simulink library "PC_Simulator_Lib"  (Simulink 8.2)
settings: Solver=ode45  StartTime=0.0  StopTime=10.0  RelTol=1e-3
values from neighbouring files (symbols this model uses):
  data = [r1 r2 r3 r4 L1 L2 L3 L4]    [strasse_Bedatung_HNI_ITI.m]
  distSameLane = 60    [InitialisationsEnv.m]
  eng_speed = [0 60 120 180 240 300 360 420 480 540 600 660 ... (101 elements, 1x101)]    [engine_table.mat]    (also in motor_parameter_calc.m = omega)
  Heading_init = 0    [Start.m]
  inertiaLateral = 25*(radiusWheel)^2    (= 4.129024)    [Start.m]
  laneWidth = 3.6    [InitialisationsEnv.m]    (also in strasse_Bedatung_HNI_ITI.m)
  omega_engine = [0.000000 150.000000 500.000000 1000.000000 1500.000000 2000.000000 2500.000000 3000.000000 3500.000000 4000.000000 4500.000000 5000.000000 5500.000000 6000.000000]    [friction_tables.m]
  omega_max = 6000    [engine_table.mat]    (also in motor_parameter_calc.m)
  omega_wheel = [0 20 40 60 80 100 122 143.7 164]    [friction_tables.m]
  para_Fellow_8_Points = ADAS.Fellow_8_Points    [ADAS_parameters.m]
  position_start_x = [x1 x2 x3 x4 x5 x6 x7]    [strasse_Bedatung_HNI_ITI.m]
  position_start_y = [y1 y2 y3 y4 y5 y6 y7]    [strasse_Bedatung_HNI_ITI.m]
  rad3rdLine = 57.2    [InitialisationsEnv.m]    (also in strasse_Bedatung_HNI_ITI.m)
  radiusWheel = 16*2.54/100    (= 0.4064)    [Start.m]
  s_values = [S1 S2 S3 S4 S5 S6 S7]    [strasse_Bedatung_HNI_ITI.m]
  segmentLimits = [segment1EndThirdLine                   segment2EndThirdLine                   segment3EndThirdLine                   segment4EndThirdLine                   segment5EndThirdLine                   segment6EndThirdLine                   segment7EndThirdLine                   segment8EndThirdLine                   ]    [InitialisationsEnv.m]    (also in strasse_Bedatung_HNI_ITI.m)
  setPosT = [-1.8 -5.4 -1.8 -5.4 -1.8 -5.4 -1.8 -5.4 -1.8 -5.4]    [InitialisationsEnv.m]
  torque = [297.089227105 300.997600937 304.800343044 308.497453426 312.088932082 315.574779014 318.95499422 322.229577701 325.398529457 328.461849487 331.419537793 334.271594373 ... (101 elements, 1x101)]    [engine_table.mat]    (also in motor_parameter_calc.m = g)
  Torque_lost = [0.000000 -8.777780 -15.000000 -26.800000 -29.600000 -32.700000 -35.900000 -39.300000 -42.800000 -46.500000 -50.300000 -54.300000 -58.500000 -62.800000 ]*0.6    [friction_tables.m]
  Torque_lost_wheel = [0.8 0.8 0.75 0.7 0.4 0.3 0.2 0.07 0.07]*0.2    [friction_tables.m]
  X_init = 0    [Start.m]
  Y_init = 1.8    [Start.m]
  Z_init = 0    [Start.m]
undefined symbols (not defined in the file or in its folder): Acc_Pedal, ADAS, Brake_Pedal, Joystick, Newton, Para, Raphson, Standard_Devices, Steering_Wheel_Angle, UDP_Protocol
libraries: simulink x43, rtwinlib x7, dspnetwork x2, simulink_extras x1, vrlib x1
(part 1 of 13)
settings Model: Creator=fahim  LastModifiedBy=fahim

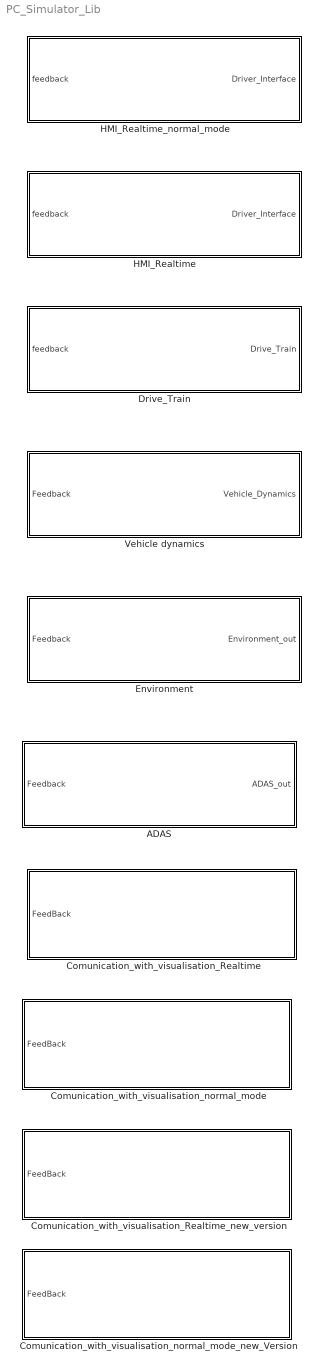
== system PC_Simulator_Lib ==
  ADAS : Subsystem
  Comunication_with_visualisation_Realtime : Subsystem
  Comunication_with_visualisation_Realtime_new_version : Subsystem
  Comunication_with_visualisation_normal_mode : Subsystem
  Comunication_with_visualisation_normal_mode_new_Version : Subsystem
  Drive_Train : Subsystem
  Environment : Subsystem
  HMI_Realtime : Subsystem
  HMI_Realtime_normal_mode : Subsystem
  Vehicle dynamics : Subsystem

== system PC_Simulator_Lib/ADAS ==
  Feedback : Inport
  Bus Creator : BusCreator  Inputs=9
  Bus Creator1 : BusCreator
  Bus Creator2 : BusCreator
  Bus Selector : BusSelector  OutputSignals=Execution_ADAS.actions_on_vehicle.Acc_Pedal[norm],Execution_ADAS.actions_on_vehicle.Brake_Pedal[norm],Execution_ADAS.actions_on_vehicle.Steering_Wheel_Angle[norm],Decision_Making_ADAS.Enable_Lateral_Controller,Unser_Interface_ADAS.ACC.ACC_Set_Speed[m|s],Decision_Making_ADAS.level_of_danger_front[0-3],Decision_Making_ADAS.Brake_distance[m],Sensors_ADAS.Sensors_Front_Out.Distance[m],Unser_Interface_ADAS.ACC.ACC_State,Unser_Interface_ADAS.Pilotiertes_Fahren.Pilotiertes_Fahren_State,Unser_Interface_ADAS.Emergency_Brake.Emergency_Brake_State,Unser_Interface_ADAS.Emergency_Steering.Emergency_Steering_State
  Decision_Making_ADAS : Subsystem
  Execution_ADAS : Subsystem
  Sensors_ADAS : Subsystem
  Unser_Interface_ADAS : Subsystem
  ADAS_out : Outport
  wires:
  Bus Selector/8 -> Bus Creator/8  "<Distance[m]>"
  Bus Selector/7 -> Bus Creator/7  "<Brake_distance[m]>"
  Bus Selector/6 -> Bus Creator/6  "<level_of_danger_front[0-3]>"
  Bus Selector/5 -> Bus Creator/5  "<ACC_Set_Speed[m|s]>"
  Bus Creator/1 -> ADAS_out/1  "ADAS"
  Unser_Interface_ADAS/1(UnserInterface_ADAS) -> Bus Creator1/1  "Unser_Interface_ADAS"
  Sensors_ADAS/1(Sensors_ADAS) -> Bus Creator1/2  "Sensors_ADAS"
  Decision_Making_ADAS/1(Decision_ADAS) -> Bus Creator1/3  "Decision_Making_ADAS"
  Execution_ADAS/1(Execution_ADAS) -> Bus Creator1/4  "Execution_ADAS"
  Bus Creator1/1 -> Sensors_ADAS/1(Feedback_ADAS), Unser_Interface_ADAS/1(Feedback_ADAS), Decision_Making_ADAS/1(Feedback_ADAS), Execution_ADAS/1(Feedback_ADAS), Bus Selector/1
  Feedback/1 -> Unser_Interface_ADAS/2(Feedback_Simulationsumgebung), Sensors_ADAS/2(Feedback_Simulationsumgebung), Execution_ADAS/2(Feedback_Simulationsumgebung), Decision_Making_ADAS/2(Feedback_Simulationsumgebung)
  Bus Selector/1 -> Bus Creator/1  "<Acc_Pedal[norm]>"
  Bus Selector/2 -> Bus Creator/2  "<Brake_Pedal[norm]>"
  Bus Selector/3 -> Bus Creator/3  "<Steering_Wheel_Angle[norm]>"
  Bus Creator2/1 -> Bus Creator/9  "ADAS_Systems_States"
  Bus Selector/9 -> Bus Creator2/1  "<ACC_State>"
  Bus Selector/10 -> Bus Creator2/2  "<Pilotiertes_Fahren_State>"
  Bus Selector/11 -> Bus Creator2/3  "<Emergency_Brake_State>"
  Bus Selector/12 -> Bus Creator2/4  "<Emergency_Steering_State>"
  Bus Selector/4 -> Bus Creator/4  "<Enable_Lateral_Controller>"

== system PC_Simulator_Lib/Comunication_with_visualisation_Realtime ==
  FeedBack : Inport
  Bus Selector : BusSelector  OutputSignals=Vehicle_Dynamics.position_CoG,Vehicle_Dynamics.Oriantation_CoG
  Bus Selector1 : BusSelector  OutputSignals=ADAS.Steering_Wheel_Angle[norm]
  Bus Selector2 : BusSelector  OutputSignals=Drive_Train.Omega_Engine[rad|s]
  Bus Selector3 : BusSelector  OutputSignals=Vehicle_Dynamics.Vx_COG[m|s]
  Embedded MATLAB Function : MATLAB Function  TreatAsAtomicUnit=on
  Gain : Gain  Gain=180/pi
  Gain1 : Gain  Gain=0.5
  Gain2 : Gain  Gain=-450
  Maping_Block : Subsystem
  Packet Output : rtwinlib/Packet Output  SampleTime=0.001  MaxMissedTicks=[]  ShowMissedTicks=off  YieldWhenWaiting=on  DrvName=Standard_Devices/UDP_Protocol  DrvAddress=15005  DrvOptions=[2213172829 15005]  PacketSize=1064  DataTypes='1064*uint8'  ShowReady=off  ShowError=off  PacketID=1  ByteOrder=1  InitialValue=[]  FinalValue=[]
      settings: AttributesFormatString=Standard Devices\nUDP Protocol [3A9Dh]
  Subsystem : Subsystem
  Subsystem1 : Subsystem
  Subsystem2 : Subsystem
  Subsystem3 : Subsystem
  Subsystem4 : Subsystem
  Subsystem5 : Subsystem
  wires:
  Embedded MATLAB Function/1(y) -> Packet Output/1
  Bus Selector/2 -> Subsystem1/1(In1)  "<Oriantation_CoG>"
  Bus Selector/1 -> Subsystem/1(In1)  "<position_CoG>"
  Subsystem/1(Out1) -> Maping_Block/1(VUT_Position_xyz[m])
  Subsystem1/1(Out1) -> Gain/1
  Subsystem2/2(Vehicle_1_Vector) -> Maping_Block/8(Vehicle_1_Vector)
  Subsystem2/3(Vehicle_2_Vector) -> Maping_Block/9(Vehicle_2_Vector)
  Subsystem2/4(Vehicle_3_Vector) -> Maping_Block/10(Vehicle_3_Vector)
  Subsystem2/5(Vehicle_4_Vector3) -> Maping_Block/11(Vehicle_4_Vector)
  Subsystem2/6(Vehicle_5_Vector) -> Maping_Block/12(Vehicle_5_Vector)
  Subsystem2/7(Vehicle_6_Vector) -> Maping_Block/13(Vehicle_6_Vector)
  Subsystem2/8(Vehicle_7_Vector) -> Maping_Block/14(Vehicle_7_Vector)
  Subsystem2/9(Vehicle_8_Vector) -> Maping_Block/15(Vehicle_8_Vector)
  Subsystem2/10(Vehicle_9_Vector) -> Maping_Block/16(Vehicle_9_Vector)
  Subsystem2/11(Vehicle_10_Vector) -> Maping_Block/17(Vehicle_10_Vector)
  Subsystem2/12(Vehicle_11_Vector) -> Maping_Block/18(Vehicle_11_Vector)
  Subsystem2/13(Vehicle_12_Vector) -> Maping_Block/19(Vehicle_12_Vector)
  Subsystem2/14(Vehicle_13_Vector) -> Maping_Block/20(Vehicle_13_Vector)
  Subsystem2/15(Vehicle_14_Vector) -> Maping_Block/21(Vehicle_14_Vector)
  Gain/1 -> Maping_Block/2(VUT_Oriantation_xyz[deg])
  Subsystem5/1(Out1) -> Maping_Block/4(VUT_Front_Wheels_Steering_Angle[deg])
  Subsystem2/1(Enablble_Fellow_Vehicles[bool]) -> Maping_Block/7(Enable_Vehicles_Vector_14[bool])
  Maping_Block/1(To_UDP) -> Embedded MATLAB Function/1(u)
  Subsystem3/1(Out1) -> Maping_Block/6(VUT_Engine_rpm)
  Bus Selector1/1 -> Gain2/1  "<Steering_Wheel_Angle[norm]>"
  Gain1/1 -> Maping_Block/3(VUT_Steering_Wheel_Angle[deg])
  Gain2/1 -> Gain1/1
  Bus Selector3/1 -> Subsystem4/1(In1)  "<Vx_COG[m|s]>"
  Subsystem4/1(Out1) -> Maping_Block/5(VUT_Wheels_Rotation_Angle[rad])
  FeedBack/1 -> Bus Selector/1, Bus Selector3/1, Bus Selector2/1, Subsystem2/1(FeedBack), Subsystem5/1(In1), Bus Selector1/1
  Bus Selector2/1 -> Subsystem3/1(In1)  "<Omega_Engine[rad|s]>"

== system PC_Simulator_Lib/Comunication_with_visualisation_Realtime_new_version ==
  FeedBack : Inport
  Bus Selector : BusSelector  OutputSignals=Vehicle_Dynamics.position_CoG,Vehicle_Dynamics.Oriantation_CoG
  Bus Selector1 : BusSelector  OutputSignals=ADAS.Steering_Wheel_Angle[norm]
  Bus Selector2 : BusSelector  OutputSignals=Drive_Train.Omega_Engine[rad|s]
  Bus Selector3 : BusSelector  OutputSignals=Vehicle_Dynamics.Vx_COG[m|s]
  Bus Selector4 : BusSelector  OutputSignals=ADAS.ACC_Set_Speed[m|s],ADAS.level_of_danger_front[0-3]
  Embedded MATLAB Function : MATLAB Function  TreatAsAtomicUnit=on
  Gain : Gain  Gain=180/pi
  Gain2 : Gain  Gain=-450
  Ground : Ground
  Ground1 : Ground
  Ground2 : Ground
  Maping_Block : Subsystem
  Packet Output : rtwinlib/Packet Output  SampleTime=0.001  MaxMissedTicks=[]  ShowMissedTicks=off  YieldWhenWaiting=on  DrvName=Standard_Devices/UDP_Protocol  DrvAddress=15005  DrvOptions=[2213172829 15005]  PacketSize=1120  DataTypes='1120*uint8'  ShowReady=off  ShowError=off  PacketID=1  ByteOrder=1  InitialValue=[]  FinalValue=[]
      settings: AttributesFormatString=Standard Devices\nUDP Protocol [3A9Dh]
  Subsystem : Subsystem
  Subsystem1 : Subsystem
  Subsystem2 : Subsystem
  Subsystem3 : Subsystem
  Subsystem4 : Subsystem
  Subsystem5 : Subsystem
  Subsystem6 : Subsystem
  scaling_factor : Gain  Gain=0.4457
  scaling_factor1 : Gain  Gain=1/8
  scaling_factor2 : Gain  Gain=3.6
  scaling_factor3 : Gain  Gain=3.6
  wires:
  scaling_factor3/1 -> Maping_Block/23(User_Set_Speed[km|h])
  Bus Selector4/2 -> Maping_Block/24(LED_Front_State)  "<level_of_danger_front[0-3]>"
  Bus Selector4/1 -> scaling_factor3/1  "<ACC_Set_Speed[m|s]>"
  Subsystem6/1(Out1) -> Maping_Block/22(Activated_ADAS)
  Ground2/1 -> Maping_Block/27(LED_Left_State)
  Ground1/1 -> Maping_Block/26(LED_Right_State)
  Ground/1 -> Maping_Block/25(LED_Back_State)
  scaling_factor2/1 -> scaling_factor/1
  scaling_factor/1 -> Maping_Block/21(VUT_Speed[km|h])
  Bus Selector2/1 -> Subsystem3/1(In1)  "<Omega_Engine[rad|s]>"
  FeedBack/1 -> Bus Selector1/1, Subsystem5/1(In1), Bus Selector3/1, Bus Selector2/1, Subsystem6/1(In1), Bus Selector4/1, Subsystem2/1(FeedBack), Bus Selector/1
  Subsystem4/1(Out1) -> Maping_Block/5(VUT_Wheels_Rotation_Angle[rad])
  Bus Selector3/1 -> Subsystem4/1(In1), scaling_factor2/1  "<Vx_COG[m|s]>"
  Gain2/1 -> scaling_factor1/1
  scaling_factor1/1 -> Maping_Block/3(VUT_Steering_Wheel_Angle[deg])
  Bus Selector1/1 -> Gain2/1  "<Steering_Wheel_Angle[norm]>"
  Subsystem3/1(Out1) -> Maping_Block/6(VUT_Engine_rpm)
  Maping_Block/1(To_UDP) -> Embedded MATLAB Function/1(u)
  Subsystem5/1(Out1) -> Maping_Block/4(VUT_Front_Wheels_Steering_Angle[deg])
  Gain/1 -> Maping_Block/2(VUT_Oriantation_xyz[deg])
  Subsystem2/14(Vehicle_14_Vector) -> Maping_Block/20(Vehicle_14_Vector)
  Subsystem2/13(Vehicle_13_Vector) -> Maping_Block/19(Vehicle_13_Vector)
  Subsystem2/12(Vehicle_12_Vector) -> Maping_Block/18(Vehicle_12_Vector)
  Subsystem2/11(Vehicle_11_Vector) -> Maping_Block/17(Vehicle_11_Vector)
  Subsystem2/10(Vehicle_10_Vector) -> Maping_Block/16(Vehicle_10_Vector)
  Subsystem2/9(Vehicle_9_Vector) -> Maping_Block/15(Vehicle_9_Vector)
  Subsystem2/8(Vehicle_8_Vector) -> Maping_Block/14(Vehicle_8_Vector)
  Subsystem2/7(Vehicle_7_Vector) -> Maping_Block/13(Vehicle_7_Vector)
  Subsystem2/6(Vehicle_6_Vector) -> Maping_Block/12(Vehicle_6_Vector)
  Subsystem2/5(Vehicle_5_Vector) -> Maping_Block/11(Vehicle_5_Vector)
  Subsystem2/4(Vehicle_4_Vector3) -> Maping_Block/10(Vehicle_4_Vector)
  Subsystem2/3(Vehicle_3_Vector) -> Maping_Block/9(Vehicle_3_Vector)
  Subsystem2/2(Vehicle_2_Vector) -> Maping_Block/8(Vehicle_2_Vector)
  Subsystem2/1(Vehicle_1_Vector) -> Maping_Block/7(Vehicle_1_Vector)
  Subsystem1/1(Out1) -> Gain/1
  Subsystem/1(Out1) -> Maping_Block/1(VUT_Position_xyz[m])
  Bus Selector/1 -> Subsystem/1(In1)  "<position_CoG>"
  Bus Selector/2 -> Subsystem1/1(In1)  "<Oriantation_CoG>"
  Embedded MATLAB Function/1(y) -> Packet Output/1

== system PC_Simulator_Lib/Comunication_with_visualisation_normal_mode ==
  FeedBack : Inport
  Bus Selector : BusSelector  OutputSignals=Vehicle_Dynamics.position_CoG,Vehicle_Dynamics.Oriantation_CoG
  Bus Selector1 : BusSelector  OutputSignals=ADAS.Steering_Wheel_Angle[norm]
  Bus Selector2 : BusSelector  OutputSignals=Drive_Train.Omega_Engine[rad|s]
  Bus Selector3 : BusSelector  OutputSignals=Vehicle_Dynamics.Vx_COG[m|s]
  Embedded MATLAB Function : MATLAB Function  TreatAsAtomicUnit=on
  Gain : Gain  Gain=180/pi
  Gain1 : Gain  Gain=0.5
  Gain2 : Gain  Gain=-450
  Maping_Block : Subsystem
  Subsystem : Subsystem
  Subsystem1 : Subsystem
  Subsystem2 : Subsystem
  Subsystem3 : Subsystem
  Subsystem4 : Subsystem
  Subsystem5 : Subsystem
  UDP Send : dspnetwork/UDP Send  remoteURL='131.234.86.93'  remotePort=15005  localURL='0.0.0.0'  localPortSource=Automatically determine  localPort=-1  sampletime=-1  separateLengthPort=0
  wires:
  Embedded MATLAB Function/1(y) -> UDP Send/1
  Bus Selector/2 -> Subsystem1/1(In1)  "<Oriantation_CoG>"
  Bus Selector/1 -> Subsystem/1(In1)  "<position_CoG>"
  Subsystem/1(Out1) -> Maping_Block/1(VUT_Position_xyz[m])
  Subsystem1/1(Out1) -> Gain/1
  Subsystem2/2(Vehicle_1_Vector) -> Maping_Block/8(Vehicle_1_Vector)
  Subsystem2/3(Vehicle_2_Vector) -> Maping_Block/9(Vehicle_2_Vector)
  Subsystem2/4(Vehicle_3_Vector) -> Maping_Block/10(Vehicle_3_Vector)
  Subsystem2/5(Vehicle_4_Vector3) -> Maping_Block/11(Vehicle_4_Vector)
  Subsystem2/6(Vehicle_5_Vector) -> Maping_Block/12(Vehicle_5_Vector)
  Subsystem2/7(Vehicle_6_Vector) -> Maping_Block/13(Vehicle_6_Vector)
  Subsystem2/8(Vehicle_7_Vector) -> Maping_Block/14(Vehicle_7_Vector)
  Subsystem2/9(Vehicle_8_Vector) -> Maping_Block/15(Vehicle_8_Vector)
  Subsystem2/10(Vehicle_9_Vector) -> Maping_Block/16(Vehicle_9_Vector)
  Subsystem2/11(Vehicle_10_Vector) -> Maping_Block/17(Vehicle_10_Vector)
  Subsystem2/12(Vehicle_11_Vector) -> Maping_Block/18(Vehicle_11_Vector)
  Subsystem2/13(Vehicle_12_Vector) -> Maping_Block/19(Vehicle_12_Vector)
  Subsystem2/14(Vehicle_13_Vector) -> Maping_Block/20(Vehicle_13_Vector)
  Subsystem2/15(Vehicle_14_Vector) -> Maping_Block/21(Vehicle_14_Vector)
  Gain/1 -> Maping_Block/2(VUT_Oriantation_xyz[deg])
  Subsystem5/1(Out1) -> Maping_Block/4(VUT_Front_Wheels_Steering_Angle[deg])
  Subsystem2/1(Enablble_Fellow_Vehicles[bool]) -> Maping_Block/7(Enable_Vehicles_Vector_14[bool])
  Maping_Block/1(To_UDP) -> Embedded MATLAB Function/1(u)
  Subsystem3/1(Out1) -> Maping_Block/6(VUT_Engine_rpm)
  Bus Selector1/1 -> Gain2/1  "<Steering_Wheel_Angle[norm]>"
  Gain1/1 -> Maping_Block/3(VUT_Steering_Wheel_Angle[deg])
  Gain2/1 -> Gain1/1
  Bus Selector3/1 -> Subsystem4/1(In1)  "<Vx_COG[m|s]>"
  Subsystem4/1(Out1) -> Maping_Block/5(VUT_Wheels_Rotation_Angle[rad])
  FeedBack/1 -> Bus Selector/1, Bus Selector3/1, Bus Selector2/1, Subsystem2/1(FeedBack), Subsystem5/1(In1), Bus Selector1/1
  Bus Selector2/1 -> Subsystem3/1(In1)  "<Omega_Engine[rad|s]>"

== system PC_Simulator_Lib/Comunication_with_visualisation_normal_mode_new_Version ==
  FeedBack : Inport
  Bus Selector : BusSelector  OutputSignals=Vehicle_Dynamics.position_CoG,Vehicle_Dynamics.Oriantation_CoG
  Bus Selector1 : BusSelector  OutputSignals=ADAS.Steering_Wheel_Angle[norm]
  Bus Selector2 : BusSelector  OutputSignals=Drive_Train.Omega_Engine[rad|s]
  Bus Selector3 : BusSelector  OutputSignals=Vehicle_Dynamics.Vx_COG[m|s]
  Bus Selector4 : BusSelector  OutputSignals=ADAS.ACC_Set_Speed[m|s],ADAS.level_of_danger_front[0-3]
  Embedded MATLAB Function : MATLAB Function  TreatAsAtomicUnit=on
  Gain : Gain  Gain=180/pi
  Gain2 : Gain  Gain=-450
  Ground : Ground
  Ground1 : Ground
  Ground2 : Ground
  Maping_Block : Subsystem
  Subsystem : Subsystem
  Subsystem1 : Subsystem
  Subsystem2 : Subsystem
  Subsystem3 : Subsystem
  Subsystem4 : Subsystem
  Subsystem5 : Subsystem
  Subsystem6 : Subsystem
  UDP Send : dspnetwork/UDP Send  remoteURL='131.234.86.93'  remotePort=15005  localURL='0.0.0.0'  localPortSource=Automatically determine  localPort=-1  sampletime=-1  separateLengthPort=0
  scaling_factor : Gain  Gain=0.4457
  scaling_factor1 : Gain  Gain=1/8
  scaling_factor2 : Gain  Gain=3.6
  scaling_factor3 : Gain  Gain=3.6
  wires:
  scaling_factor3/1 -> Maping_Block/23(User_Set_Speed[km|h])
  Bus Selector4/2 -> Maping_Block/24(LED_Front_State)  "<level_of_danger_front[0-3]>"
  Bus Selector4/1 -> scaling_factor3/1  "<ACC_Set_Speed[m|s]>"
  Subsystem6/1(Out1) -> Maping_Block/22(Activated_ADAS)
  Ground2/1 -> Maping_Block/27(LED_Left_State)
  Ground1/1 -> Maping_Block/26(LED_Right_State)
  Ground/1 -> Maping_Block/25(LED_Back_State)
  scaling_factor2/1 -> scaling_factor/1
  scaling_factor/1 -> Maping_Block/21(VUT_Speed[km|h])
  Bus Selector2/1 -> Subsystem3/1(In1)  "<Omega_Engine[rad|s]>"
  FeedBack/1 -> Bus Selector1/1, Subsystem5/1(In1), Bus Selector3/1, Bus Selector2/1, Subsystem6/1(In1), Bus Selector4/1, Subsystem2/1(FeedBack), Bus Selector/1
  Subsystem4/1(Out1) -> Maping_Block/5(VUT_Wheels_Rotation_Angle[rad])
  Bus Selector3/1 -> Subsystem4/1(In1), scaling_factor2/1  "<Vx_COG[m|s]>"
  Gain2/1 -> scaling_factor1/1
  scaling_factor1/1 -> Maping_Block/3(VUT_Steering_Wheel_Angle[deg])
  Bus Selector1/1 -> Gain2/1  "<Steering_Wheel_Angle[norm]>"
  Subsystem3/1(Out1) -> Maping_Block/6(VUT_Engine_rpm)
  Maping_Block/1(To_UDP) -> Embedded MATLAB Function/1(u)
  Subsystem5/1(Out1) -> Maping_Block/4(VUT_Front_Wheels_Steering_Angle[deg])
  Gain/1 -> Maping_Block/2(VUT_Oriantation_xyz[deg])
  Subsystem2/14(Vehicle_14_Vector) -> Maping_Block/20(Vehicle_14_Vector)
  Subsystem2/13(Vehicle_13_Vector) -> Maping_Block/19(Vehicle_13_Vector)
  Subsystem2/12(Vehicle_12_Vector) -> Maping_Block/18(Vehicle_12_Vector)
  Subsystem2/11(Vehicle_11_Vector) -> Maping_Block/17(Vehicle_11_Vector)
  Subsystem2/10(Vehicle_10_Vector) -> Maping_Block/16(Vehicle_10_Vector)
  Subsystem2/9(Vehicle_9_Vector) -> Maping_Block/15(Vehicle_9_Vector)
  Subsystem2/8(Vehicle_8_Vector) -> Maping_Block/14(Vehicle_8_Vector)
  Subsystem2/7(Vehicle_7_Vector) -> Maping_Block/13(Vehicle_7_Vector)
  Subsystem2/6(Vehicle_6_Vector) -> Maping_Block/12(Vehicle_6_Vector)
  Subsystem2/5(Vehicle_5_Vector) -> Maping_Block/11(Vehicle_5_Vector)
  Subsystem2/4(Vehicle_4_Vector3) -> Maping_Block/10(Vehicle_4_Vector)
  Subsystem2/3(Vehicle_3_Vector) -> Maping_Block/9(Vehicle_3_Vector)
  Subsystem2/2(Vehicle_2_Vector) -> Maping_Block/8(Vehicle_2_Vector)
  Subsystem2/1(Vehicle_1_Vector) -> Maping_Block/7(Vehicle_1_Vector)
  Subsystem1/1(Out1) -> Gain/1
  Subsystem/1(Out1) -> Maping_Block/1(VUT_Position_xyz[m])
  Bus Selector/1 -> Subsystem/1(In1)  "<position_CoG>"
  Bus Selector/2 -> Subsystem1/1(In1)  "<Oriantation_CoG>"
  Embedded MATLAB Function/1(y) -> UDP Send/1

== system PC_Simulator_Lib/Drive_Train ==
  feedback : Inport
  4_Wheels_drive_train_and_Brake : Subsystem
  Bus Selector : BusSelector  OutputSignals=Vehicle_Dynamics.Vx_COG[m|s],Driver_Interface.DNR
  Bus Selector1 : BusSelector  OutputSignals=ADAS.Acc_Pedal[norm]
  Differential : Subsystem
  Engine : Subsystem
  Gain : Gain  Gain=3.6
  Gearbox : Subsystem
  Mux2 : Mux  Inputs=2
  Mux3 : Mux  Inputs=2
  Output_Interface : Subsystem
  Drive_Train : Outport
  wires:
  Output_Interface/1(Drive_Train) -> Drive_Train/1
  feedback/1 -> 4_Wheels_drive_train_and_Brake/1(Feedback), Bus Selector/1, Bus Selector1/1
  Bus Selector/1 -> Gain/1  "<Vx_COG[m|s]>"
  Gain/1 -> Gearbox/1(velocity)
  Bus Selector/2 -> Gearbox/2(DNR)  "<DNR>"
  Engine/1(Torque) -> Gearbox/3(Torque_Engine)
  Gearbox/1(omega_engine_radPs) -> Engine/2(Omega_engine_radPs), Output_Interface/13(Omega_Engine[rad|s])
  Gearbox/2(Torque_out_gearbox_Nm) -> Differential/1(Torque_in)
  Differential/3(omega_out_gearbox_radPs) -> Gearbox/4(omega_out_gearbox_radPs)
  Differential/4(omegaDot_out_gearbox_radPs1) -> Gearbox/5(omegaDot_out_gearbox_radPs2)
  Differential/1(Torque_out_1) -> 4_Wheels_drive_train_and_Brake/2(Torque_RL[Nm])
  Differential/2(Torque_out_2) -> 4_Wheels_drive_train_and_Brake/3(Torque_RR[Nm])
  4_Wheels_drive_train_and_Brake/11(Omega_RL[rad|s]) -> Mux2/1, Output_Interface/11(Omega_RL[rad|s])
  4_Wheels_drive_train_and_Brake/12(OmegaDot_RL[rad|s^2]) -> Mux2/2
  4_Wheels_drive_train_and_Brake/13(Omega_RR[rad|s]) -> Mux3/1, Output_Interface/12(Omega_RR[rad|s])
  4_Wheels_drive_train_and_Brake/14(OmegaDot_RR[rad|s^2]) -> Mux3/2
  Mux2/1 -> Differential/2(rotation_1)
  Mux3/1 -> Differential/3(rotation_2)
  Gearbox/3(omegaDot_engine_radPs2) -> Engine/3(OmegaDot_engine_radPs2)
  4_Wheels_drive_train_and_Brake/1(Fx_FL[N]) -> Output_Interface/1(Force_tire_x_FL[N])
  4_Wheels_drive_train_and_Brake/2(Fx_FR[N]) -> Output_Interface/2(Force_tire_x_FR[N])
  4_Wheels_drive_train_and_Brake/3(Fx_RL[N]) -> Output_Interface/3(Force_tire_x_RL[N])
  4_Wheels_drive_train_and_Brake/4(Fx_RR[N]) -> Output_Interface/4(Force_tire_x_RR[N])
  4_Wheels_drive_train_and_Brake/5(Fy_FL[N]) -> Output_Interface/5(Force_tire_y_FL[N])  "Force_tire_y_FL_N"
  4_Wheels_drive_train_and_Brake/6(Fy_FR[N]) -> Output_Interface/6(Force_tire_y_FR[N])  "Force_tire_y_FR_N"
  4_Wheels_drive_train_and_Brake/7(Fy_RL[N]) -> Output_Interface/7(Force_tire_y_RL[N])  "Force_tire_y_RL_N"
  4_Wheels_drive_train_and_Brake/8(Fy_RR[N]) -> Output_Interface/8(Force_tire_y_RR[N])  "Force_tire_y_RR_N"
  4_Wheels_drive_train_and_Brake/9(Omega_FL[rad|s]) -> Output_Interface/9(Omega_FL[rad|s])
  4_Wheels_drive_train_and_Brake/10(Omega_FR[rad|s]) -> Output_Interface/10(Omega_FR[rad|s])
  Gearbox/4(Gearbox_Gear_Ratio) -> Output_Interface/14(Gearbox_Gear_Ratio)
  Bus Selector1/1 -> Engine/1(Throttle)  "<Acc_Pedal[norm]>"

== system PC_Simulator_Lib/Environment ==
  Feedback : Inport
  Environment_Model : Subsystem
  "Maping_Input " : Subsystem
  "Maping_Output " : Subsystem
  Environment_out : Outport
  wires:
  "Maping_Output "/1(Out1) -> Environment_out/1
  Environment_Model/1(x_fellows_Vector[m]) -> "Maping_Output "/1(x_fellows_Vector[m])
  Environment_Model/2(y_fellows_Vector[m]) -> "Maping_Output "/2(y_fellows_Vector[m])
  Environment_Model/3(z_fellows_Vector[m]) -> "Maping_Output "/3(z_fellows_Vector[m])
  Environment_Model/4(Heading_fellows_Vector[deg]) -> "Maping_Output "/4(Heading_fellows_Vector[deg])
  Feedback/1 -> "Maping_Input "/1(Feedback)
  "Maping_Input "/2(mainCarPosT[m]) -> "Maping_Output "/6(T_VUT[m]), Environment_Model/2(mainCarPosT[m])
  "Maping_Input "/3(mainCarVelS[m/s]) -> Environment_Model/3(mainCarVelS[m/s])
  "Maping_Input "/1(mainCarPosS[m]) -> Environment_Model/1(mainCarPosS[m])
  Environment_Model/5(S_Velocity_Vector[m|s]) -> "Maping_Output "/5(S_Velocity_Vector[m|s])
  "Maping_Input "/4(Heating_Angle_Road_under_VUT[deg]) -> "Maping_Output "/7(Heating_Angle_Road_under_VUT[deg])

== system PC_Simulator_Lib/HMI_Realtime ==
  note: D..1
      | N..0
      | R..-1
  feedback : Inport
  Bus Selector : BusSelector  OutputSignals=ADAS.Steering_Wheel_Angle[norm]
  Bus Selector1 : BusSelector  OutputSignals=ADAS.Enable_Lateral_Controller
  Gain3 : Gain  Gain=450
  Gain4 : Gain  Gain=450
  HMI_Logitech1 : Subsystem
  Maping_Output : Subsystem
  Terminator{3..7} (5 alike) : Terminator
  steering wheel controller : Subsystem
  Driver_Interface : Outport
  wires:
  HMI_Logitech1/3(Brack_pedal) -> Maping_Output/3(Brake_Pedal_norm)  "Brake_Pedal_norm"
  HMI_Logitech1/2(Acceleration_pedal) -> Maping_Output/2(Acc_Pedal_norm)  "Acc_Pedal_norm"
  HMI_Logitech1/1(Steering_Wheel_norm) -> Gain4/1, Maping_Output/1(Steering_wheel_norm)  "Steering_wheel_norm"
  Gain4/1 -> steering wheel controller/1(wheel_angle_actual_deg[-450 450])
  Gain3/1 -> steering wheel controller/2(wheel_angle_desired_deg[-450 450])
  feedback/1 -> Bus Selector/1, Bus Selector1/1
  Bus Selector/1 -> Gain3/1  "<Steering_Wheel_Angle[norm]>"
  HMI_Logitech1/4(Button_1) -> Maping_Output/4(ACC_Plus)
  HMI_Logitech1/5(Button_2) -> Maping_Output/5(ACC_Minus)
  HMI_Logitech1/6(Button_3) -> Maping_Output/6(ACC_Stop)
  HMI_Logitech1/7(Button_4) -> Maping_Output/7(ACC_Resume)
  HMI_Logitech1/17(DNR) -> Maping_Output/12(DNR)  "DNR"
  Maping_Output/1(Out1) -> Driver_Interface/1
  HMI_Logitech1/10(Button_5) -> Maping_Output/10(Time_Gap_Mode_Switching)
  HMI_Logitech1/9(Left_Padel) -> Maping_Output/9(Pilot_Button)
  HMI_Logitech1/8(Right_Padel) -> Maping_Output/8(Emergency_Brake_Button)
  HMI_Logitech1/12(Button_7) -> Terminator3/1
  HMI_Logitech1/13(Button_8) -> Terminator4/1
  HMI_Logitech1/14(Button_9) -> Terminator5/1
  HMI_Logitech1/15(Button_10) -> Terminator6/1
  HMI_Logitech1/16(arrow_deg) -> Terminator7/1
  steering wheel controller/1(Out1) -> HMI_Logitech1/1(Force_Feedback)
  HMI_Logitech1/11(Button_6) -> Maping_Output/11(Emergency_Steering_Button)
  Bus Selector1/1 -> steering wheel controller/3(controller_mod)  "<Enable_Lateral_Controller>"

== system PC_Simulator_Lib/HMI_Realtime_normal_mode ==
  note: D..1
      | N..0
      | R..-1
  feedback : Inport
  HMI_Logitech : Subsystem
  Maping_Output : Subsystem
  Terminator{,3..7} (6 alike) : Terminator
  Driver_Interface : Outport
  wires:
  HMI_Logitech/3(Brack_pedal) -> Maping_Output/3(Brake_Pedal_norm)  "Brake_Pedal_norm"
  HMI_Logitech/1(Steering_Wheel_norm) -> Maping_Output/1(Steering_wheel_norm)  "Steering_wheel_norm"
  HMI_Logitech/2(Acceleration_pedal) -> Maping_Output/2(Acc_Pedal_norm)  "Acc_Pedal_norm"
  feedback/1 -> Terminator/1
  HMI_Logitech/4(Button_1) -> Maping_Output/4(ACC_Plus)
  HMI_Logitech/5(Button_2) -> Maping_Output/5(ACC_Minus)
  HMI_Logitech/6(Button_3) -> Maping_Output/6(ACC_Stop)
  HMI_Logitech/7(Button_4) -> Maping_Output/7(ACC_Resume)
  HMI_Logitech/17(DNR) -> Maping_Output/12(DNR)  "DNR"
  Maping_Output/1(Out1) -> Driver_Interface/1
  HMI_Logitech/10(Button_5) -> Maping_Output/10(Time_Gap_Mode_Switching)
  HMI_Logitech/9(Left_Padel) -> Maping_Output/9(Pilot_Button)
  HMI_Logitech/8(Right_Padel) -> Maping_Output/8(Emergency_Brake_Button)
  HMI_Logitech/12(Button_7) -> Terminator3/1
  HMI_Logitech/13(Button_8) -> Terminator4/1
  HMI_Logitech/14(Button_9) -> Terminator5/1
  HMI_Logitech/15(Button_10) -> Terminator6/1
  HMI_Logitech/16(arrow_deg) -> Terminator7/1
  HMI_Logitech/11(Button_6) -> Maping_Output/11(Emergency_Steering_Button)

== system PC_Simulator_Lib/Vehicle dynamics ==
  Feedback : Inport
  Add : Sum
  Bus Creator : BusCreator  Inputs=3
  Bus Creator1 : BusCreator  Inputs=3
  Bus Selector1 : BusSelector  OutputSignals=Force_tire_x_FL[N],Force_tire_x_FR[N],Force_tire_x_RL[N],Force_tire_x_RR[N]
  Bus Selector2 : BusSelector  OutputSignals=Force_tire_y_FL[N],Force_tire_y_FR[N],Force_tire_y_RL[N],Force_tire_y_RR[N]
  Bus Selector6 : BusSelector  OutputSignals=ADAS.Steering_Wheel_Angle[norm],Drive_Train.Force_x_tire[N],Drive_Train.Force_y_tire[N]
  Constant : Constant  Value=Z_init
  Forces_transformation : Subsystem
  Gain1 : Gain  Gain=3.6
  Ground{,1..4} (5 alike) : Ground
  Horizontal_Dyn : Subsystem
  Mux : Mux
  Output_Maping : Subsystem
  Scope : Scope
      settings: TimeRange=1.302659975172148  YMin=3  YMax=3  SaveName=ScopeData5
  Terminator{,1..7} (8 alike) : Terminator
  Vertical_Dyn. : Subsystem
  Z1(4) : Terminator
  Z1(4)1 : Terminator
  force_from_wheel_cordination_transformation : Subsystem
  velocity : Subsystem
  xy_Global : Subsystem
  Vehicle_Dynamics : Outport
  wires:
  Horizontal_Dyn/1(Longitudinal_velocity_Vx) -> Horizontal_Dyn/4(vx[m|s]), velocity/1(longitudenal_velocity_Vx), Output_Maping/4(Vx_COG[m|s]), Gain1/1, xy_Global/1(Vx_CG)  "Vx_COG[m|s]"
  Horizontal_Dyn/2(Lateral_velocity_Vy_relative_to_car) -> xy_Global/2(Vy_CG), Output_Maping/5(Vy_COG[m|s]), velocity/2(Lateral_velocity_Vy)  "Vy"
  Horizontal_Dyn/6(Beta_Slip_Angle) -> Terminator2/1, Forces_transformation/2(Slip_angle_of_velocity)
  Horizontal_Dyn/5(Displacement_x_relative_to_car) -> Terminator1/1
  Horizontal_Dyn/4(Displacement_y_relative_to_car) -> Terminator/1
  Horizontal_Dyn/7(ACC_x_relative_to_car) -> Output_Maping/6(ax_COG[m|s2])
  Horizontal_Dyn/8(ACC_Y_relative_to_car) -> Terminator4/1
  Horizontal_Dyn/9(Yaw_rate_of_change) -> Output_Maping/11(Yaw_Rate[rad|s]), velocity/3(rate_of_change_Yaw_Angle), xy_Global/3(rate_of_change_Yaw_Angle)  "Yaw_rate_of_change"
  force_from_wheel_cordination_transformation/3(angle_of_rotation_of_front_left_wheel) -> Output_Maping/12(Wheel_Steering_Angle_Left[rad]), velocity/4(angel_of_rotation_of_front_left_wheel), Output_Maping/7(Wheel_FL_Steering_Angle[rad])  "Angle_front_left_wheel"
  force_from_wheel_cordination_transformation/4(angle_of_rotation_of_front_right_wheel) -> Output_Maping/13(Wheel_Steering_Angle_Right[rad]), velocity/5(angel_of_rotation_of_front_Right_wheel), Output_Maping/8(Wheel_FR_Steering_Angle[rad])  "Angle_front_right_wheel"
  Horizontal_Dyn/10(absolute_velocity_of_car) -> Forces_transformation/1(velocity_of_car_absolute)
  force_from_wheel_cordination_transformation/1(Forces_on_x_from_wheel_mux(4)) -> Forces_transformation/3(Forces_on_x_from_wheel_mux(4))
  force_from_wheel_cordination_transformation/2(Forces_on_y_from_wheel_mux(4)) -> Forces_transformation/4(Forces_on_y_from_wheel_mux(4))
  Vertical_Dyn./5(Force_Suspention(4)) -> Forces_transformation/5(Forces_on_z_from_wheel_mux(4)), Output_Maping/3(Force_Suspention)  "Force_Suspention"
  Forces_transformation/1(Force_acting_on_CG_in_x) -> Horizontal_Dyn/1(Force_acting_on_CG_in_x)
  Forces_transformation/2(Force_acting_on_CG_in_Y) -> Horizontal_Dyn/2(Force_acting_on_CG_in_y)
  Forces_transformation/3(Moment _about _Z_axis) -> Horizontal_Dyn/3(Moment _about _Z_axis)
  Forces_transformation/4(Force_acting_on_CG_in_z) -> Vertical_Dyn./1(Vertical_Force_CG)
  Forces_transformation/5(Moment _about _X_axis) -> Vertical_Dyn./2(Moment_X-axis_CG)
  Forces_transformation/6(Moment _about _Y_axis) -> Vertical_Dyn./3(Moment_Y-axis_CG)
  Vertical_Dyn./6(Length_Suspention(4)) -> Forces_transformation/6(Length_suspention(4))
  Bus Selector1/1 -> force_from_wheel_cordination_transformation/2(force_from_wheel_fornt_left_in_x_relative_to_tire)  "<Force_tire_x_FL[N]>"
  Bus Selector1/2 -> force_from_wheel_cordination_transformation/3(force_from_wheel_fornt_right_in_x_relative_to_tire)  "<Force_tire_x_FR[N]>"
  Bus Selector1/3 -> force_from_wheel_cordination_transformation/4(force_from_wheel_rear_left_in_x_relative_to_tire)  "<Force_tire_x_RL[N]>"
  Bus Selector1/4 -> force_from_wheel_cordination_transformation/5(force_from_wheel_rear_right_in_x_relative_to_tire)  "<Force_tire_x_RR[N]>"
  Vertical_Dyn./3(pitch) -> Bus Creator/1  "Pitch_Angle"
  Vertical_Dyn./4(Roll) -> Bus Creator/2  "Roll_Angle"
  Vertical_Dyn./2(Vertical_Displacement_Z_vehicle_corners(4)) -> Terminator7/1
  Vertical_Dyn./7(Z1(4)) -> Z1(4)/1
  velocity/1(velocity_at_wheels_in_X_mux(4)) -> Output_Maping/1(Velocity_Wheels_X[m|s])  "Velocity_Wheels_X"
  velocity/2(velocity_at_wheels_in_Y_mux(4)) -> Output_Maping/2(Velocity_Wheels_Y[m|s])  "Velocity_Wheels_Y"
  Forces_transformation/7(Mass*gravity_in_Z) -> Vertical_Dyn./4(Mass*gravity_in_Z)
  Horizontal_Dyn/3("yaw ") -> Bus Creator/3, Terminator6/1  "Yaw_Angle"
  Feedback/1 -> Bus Selector6/1
  Bus Selector6/2 -> Bus Selector1/1  "<Force_x_tire[N]>"
  Gain1/1 -> Scope/1
  Bus Selector6/1 -> force_from_wheel_cordination_transformation/1(steering_Angle_HMI_in_range[-1 1])  "<Steering_Wheel_Angle[norm]>"
  xy_Global/3(x_CG) -> Bus Creator1/1  "x_CoG[m]"
  xy_Global/4(y_CG) -> Bus Creator1/2  "y_CoG[m]"
  Output_Maping/1(Vehicle_Dynamics) -> Vehicle_Dynamics/1
  Vertical_Dyn./1(Vertical_Displacement_Z_CG) -> Add/2  "Vz"
  Add/1 -> Bus Creator1/3  "z_CoG[m]"
  Constant/1 -> Add/1
  Bus Creator1/1 -> Output_Maping/9(position_CoG_Global_Vector[m])  "position_CoG"
  Bus Creator/1 -> Output_Maping/10(Oriantation_CoG_Vector[rad])  "Oriantation_CoG"
  Bus Selector6/3 -> Bus Selector2/1  "<Force_y_tire[N]>"
  Bus Selector2/1 -> force_from_wheel_cordination_transformation/6(force_from_wheel_fornt_left_in_y_relative_to_tire)  "<Force_tire_y_FL[N]>"
  Bus Selector2/2 -> force_from_wheel_cordination_transformation/7(force_from_wheel_fornt_right_in_y_relative_to_tire)  "<Force_tire_y_FR[N]>"
  Bus Selector2/3 -> force_from_wheel_cordination_transformation/8(force_from_wheel_rear_left_in_y_relative_to_tire)  "<Force_tire_y_RL[N]>"
  Bus Selector2/4 -> force_from_wheel_cordination_transformation/9(force_from_wheel_rear_right_in_y_relative_to_tire)  "<Force_tire_y_RR[N]>"
  velocity/3(R_CG) -> Terminator3/1
  Vertical_Dyn./8(Vertical_Velocity_Z_CG[m|s]) -> Z1(4)1/1
  Ground/1 -> Vertical_Dyn./5(Z0)
  Mux/1 -> Forces_transformation/7(Z0_mux(4))
  Ground1/1 -> Mux/1
  Ground2/1 -> Mux/2
  Ground3/1 -> Mux/3
  Ground4/1 -> Mux/4
  xy_Global/5(Actual_YAW) -> Terminator5/1

== system PC_Simulator_Lib/ADAS/Decision_Making_ADAS ==
  Feedback_ADAS : Inport
  Feedback_Simulationsumgebung : Inport  Port=2
  Bus Creator : BusCreator  Inputs=8
  Decision_Unit : Subsystem
  Display2 : Display
  Gain : Gain  Gain=3.6
  Maping_Input : Subsystem
  Trajectory_calculatin_and_distance_control_and output_maping : Subsystem
  Decision_ADAS : Outport
  wires:
  Decision_Unit/1(Enable_Longitudinal_Controller[bool]) -> Trajectory_calculatin_and_distance_control_and output_maping/5(Enable_Longitudinal_Control)
  Maping_Input/5(Active_System) -> Decision_Unit/1(Active_System)
  Trajectory_calculatin_and_distance_control_and output_maping/8(Brake_distance[m]1) -> Bus Creator/8
  Decision_Unit/13(Brake_distance[m]) -> Trajectory_calculatin_and_distance_control_and output_maping/17(Brake_distance[m])
  Decision_Unit/12(level_of_danger_front[0-3]) -> Trajectory_calculatin_and_distance_control_and output_maping/16(level_of_danger_front[0-3])
  Trajectory_calculatin_and_distance_control_and output_maping/7(level_of_danger_front[0-3]1) -> Bus Creator/7
  Decision_Unit/11(a_x_desiredm|s2]) -> Trajectory_calculatin_and_distance_control_and output_maping/15(a_x_desiredm|s2])
  Maping_Input/14(Heading_Angle_Difference_Absolute[deg]) -> Decision_Unit/10(Heading_Angle_Difference_absolute[deg])
  Decision_Unit/8(T_desird[m]) -> Trajectory_calculatin_and_distance_control_and output_maping/12(T_Desired_initial[m])
  Bus Creator/1 -> Decision_ADAS/1
  Feedback_ADAS/1 -> Maping_Input/1(Feedback_ADAS)
  Feedback_Simulationsumgebung/1 -> Maping_Input/2(Feedback_Simulationsumgebung)
  Trajectory_calculatin_and_distance_control_and output_maping/1(Enable_Longitudinal_Control[bool]) -> Bus Creator/1
  Trajectory_calculatin_and_distance_control_and output_maping/2(Enable_Lateral_Controller[bool]) -> Bus Creator/2
  Trajectory_calculatin_and_distance_control_and output_maping/3(Desired_Track_Bus) -> Bus Creator/3
  Trajectory_calculatin_and_distance_control_and output_maping/4(ADAS_Parameters_Bus) -> Bus Creator/4
  Maping_Input/4(Vx_CoG_VUT[m|s]) -> Gain/1, Trajectory_calculatin_and_distance_control_and output_maping/4(Vx_CoG[m|s]), Decision_Unit/11(velocity_VUT[m|s])
  Maping_Input/3(yaw_VUT[rad]) -> Trajectory_calculatin_and_distance_control_and output_maping/3(Yaw_Angle[rad])
  Maping_Input/2(y_CoG_VUT[m]) -> Trajectory_calculatin_and_distance_control_and output_maping/2(y[m])
  Maping_Input/1(x_CoG_VUT[m]) -> Trajectory_calculatin_and_distance_control_and output_maping/1(x[m])
  Maping_Input/7(Time_Gap[s]) -> Decision_Unit/3(Time_Gap_User[s])
  Decision_Unit/2(Enable_Lateral_Controller[bool]) -> Trajectory_calculatin_and_distance_control_and output_maping/6(Enable_Lateral_Controller)
  Decision_Unit/3(Velocity_desired_Free_Driving[m|s]) -> Trajectory_calculatin_and_distance_control_and output_maping/7(V_User_Set_Speed[m|s])
  Decision_Unit/4(Object_in_Lane[bool]) -> Trajectory_calculatin_and_distance_control_and output_maping/8(Enable_Distance_Control[bool])
  Decision_Unit/5(Distance_2_Object[m]) -> Trajectory_calculatin_and_distance_control_and output_maping/9(Distance_2_Felow_Vehicle[m])
  Decision_Unit/6(v_relative[m|s]) -> Trajectory_calculatin_and_distance_control_and output_maping/10(V_realtive[m|s])
  Decision_Unit/7(Time_Gap[s]) -> Trajectory_calculatin_and_distance_control_and output_maping/11(Time_Gap[s])
  Decision_Unit/9(Lateral_Velocity_Max[m|s]) -> Trajectory_calculatin_and_distance_control_and output_maping/13(Delta_T_Rate_limitl[m|s])
  Maping_Input/10(v_relative_Sensor[m|s]) -> Decision_Unit/6(v_relative_Sensor[m|s])
  Maping_Input/8(Object_Inlane[bool]) -> Decision_Unit/4(Object_Inlane[bool])
  Maping_Input/9(Distance_2_Object_Sensor[m]) -> Decision_Unit/5(Distance_2_Object_Sensor[m])
  Maping_Input/11(T_current[m]) -> Decision_Unit/7(T_current[m])
  Decision_Unit/10(Acceleration_Velocity_Control_Switching[0 1]) -> Trajectory_calculatin_and_distance_control_and output_maping/14(Acceleration_Velocity_Control_Switching[0 1])
  Trajectory_calculatin_and_distance_control_and output_maping/6("a_x_desiredm|s2]1 ") -> Bus Creator/6
  Trajectory_calculatin_and_distance_control_and output_maping/5(Acceleration_Velocity_Control_Switching[0 1]1) -> Bus Creator/5
  Maping_Input/6(V_User_Set_Speed[m|s]) -> Decision_Unit/2(Set_Speed_User[m|s])
  Gain/1 -> Display2/1
  Maping_Input/12(Direction_delta_T_Available) -> Decision_Unit/8(Direction_delta_T_Available)
  Maping_Input/13(Lateral_Distance_Available[m]) -> Decision_Unit/9(Lateral_Distance_Available[m])

== system PC_Simulator_Lib/ADAS/Execution_ADAS ==
  Feedback_ADAS : Inport
  Feedback_Simulationsumgebung : Inport  Port=2
  Input_Interface : Subsystem
  Lateral_Controller_S_Function : Subsystem
  Longitudinal_Controller : Subsystem
  Output_Interface : Subsystem
  Execution_ADAS : Outport
  wires:
  Feedback_ADAS/1 -> Input_Interface/1(Feedback_ADAS)
  Feedback_Simulationsumgebung/1 -> Input_Interface/2(Feedback_Simulationsumgebung)
  Input_Interface/1(a_x_actual[m|s2]) -> Longitudinal_Controller/2(a_acctual[m|s2])
  Input_Interface/3(Omega_4_Wheels[rad|s]) -> Longitudinal_Controller/4(omega_4_Wheels[rad|s])
  Input_Interface/4(Omega_Engine[rad|s]) -> Longitudinal_Controller/5(Omega_Engine[rad|s])
  Input_Interface/5(Gearbox_Gear_Ratio) -> Longitudinal_Controller/6(Gearbox_Gear_Ratio)
  Input_Interface/6(Differential_Gear_Ratio) -> Longitudinal_Controller/7(Differential_Gear_Ratio)
  Longitudinal_Controller/1(Acc_Pedal[norm]) -> Output_Interface/1(Acc_Pedal[norm])  "Acc_Pedal[norm]"
  Longitudinal_Controller/2(Brake_Pedal[norm]) -> Output_Interface/2(Brake_Pedal[norm])  "Brake_Pedal[norm]"
  Input_Interface/11(Eanbel_Longitudidinal_Controller) -> Longitudinal_Controller/Enable, Output_Interface/3(Eanbel_Longitudidinal_Controller)
  Input_Interface/13(Acc_Pedal_user[norm]) -> Output_Interface/5(Acc_Pedal_user[norm])
  Input_Interface/14(Brake_Pedal_user[norm]) -> Output_Interface/6(Brake_Pedal_user[norm])
  Output_Interface/1(Out1) -> Execution_ADAS/1
  Input_Interface/15(Steering_Wheel_Angle[norm]) -> Output_Interface/8(Steering_Wheel_Angle_User[norm])
  Input_Interface/20(y_CoG[m]) -> Lateral_Controller_S_Function/6(y_CoG[m])
  Input_Interface/19(x_CoG[m]) -> Lateral_Controller_S_Function/5(x_CoG[m])
  Input_Interface/18(Yaw_Rate[rad|s]) -> Lateral_Controller_S_Function/4(Yaw_Rate[rad|s])
  Input_Interface/17(Yaw_Angle[rad]) -> Lateral_Controller_S_Function/3(Yaw_Angle[rad])
  Input_Interface/16(Vy_CoG[m|s]) -> Lateral_Controller_S_Function/2(Vy_CoG[m|s])
  Input_Interface/21(x_Desired[m]) -> Lateral_Controller_S_Function/7(x_Desired[m])
  Input_Interface/22(y_Desired[m]) -> Lateral_Controller_S_Function/8(y_Desired[m])
  Input_Interface/26(Curvature_Desired_Track[1|m]) -> Lateral_Controller_S_Function/12(Curvature_Desired_Track[1|m])
  Input_Interface/24(acceleration_Desired[m|s2]) -> Lateral_Controller_S_Function/10(acceleration_Desired[m|s2])
  Input_Interface/25(Heading_Angle_Desired[rad]) -> Lateral_Controller_S_Function/11(Heading_Angle_Desired[rad])
  Input_Interface/23(Velocity_Desired[m|s]) -> Longitudinal_Controller/1(Vx_desired[m|s]), Lateral_Controller_S_Function/9(Velocity_Desired[m|s])
  Input_Interface/2(Vx_CoG[m|s]) -> Lateral_Controller_S_Function/1(Vx_CoG[m|s]), Longitudinal_Controller/3(Vx_CoG[m|s])
  Lateral_Controller_S_Function/1(Steering_Wheel_Angle[norm]) -> Output_Interface/7(Steering_Wheel_Angle_Controller[norm])
  Input_Interface/12(Eanbel_Lateral_Controller) -> Lateral_Controller_S_Function/Enable, Output_Interface/4(Eanbel_Lateral_Controller)
  Input_Interface/8(acceleration_min[m|s2]) -> Longitudinal_Controller/9(acceleration_min[m|s2])
  Input_Interface/7(acceleration_max[m|s2]) -> Longitudinal_Controller/8(acceleration_max[m|s2])
  Input_Interface/9(Acceleration_Velocity_Control_Switching[0 1]) -> Longitudinal_Controller/10(Acceleration_Velocity_Control_Switching[0|1])
  Input_Interface/10(a_x_desired[m|s2]) -> Longitudinal_Controller/11(ax_desired[m|s2])

== system PC_Simulator_Lib/ADAS/Sensors_ADAS ==
  Feedback_ADAS : Inport
  Feedback_Simulationsumgebung : Inport  Port=2
  Bus Selector : BusSelector  OutputSignals=Environment.Main_Vehicle.Heating_Angle_Road_under_VUT[deg],Vehicle_Dynamics.Oriantation_CoG.Yaw_Angle
  Front_Long_Range_Radar_Sensor : Subsystem  mask{para_num_fellow=ADAS.Num_Fellows, para_filter_radius=ADAS.Front_Long_Range_Radar.filter_radius, LocPosTriang=ADAS.Front_Long_Range_Radar}
      mask prompts: para_num_fellow "Number of Fellow Objects"; para_filter_radius "Sphere Filter Radius"; LocPosTriang "Local Position of the Radar Triangles"
      mask DialogControl DescTextVar Prompt: a general radar sensor model
  Front_Mid_Range_Radar_Sensor : Subsystem  mask{para_num_fellow=ADAS.Num_Fellows, para_filter_radius=ADAS.Front_Mid_Range_Radar.filter_radius, LocPosTriang=ADAS.Front_Mid_Range_Radar}
      mask prompts: para_num_fellow "Number of Fellow Objects"; para_filter_radius "Sphere Filter Radius"; LocPosTriang "Local Position of the Radar Triangles"
      mask DialogControl DescTextVar Prompt: a general radar sensor model
  Input_Maping : Subsystem
  Object_Selection_Based_On_LRR_MRR_and_Camera SENSOR FUSION : Subsystem
  Output_Mapint : Subsystem
  convert_xy_2_st : Subsystem  mask{para_num_fellow=ADAS.Num_Fellows}
      mask prompts: para_num_fellow "Number of Fellow Objects"
  convert_xy_2_st1 : Subsystem  mask{para_num_fellow=ADAS.Num_Fellows}
      mask prompts: para_num_fellow "Number of Fellow Objects"
  Sensors_ADAS : Outport
  wires:
  Front_Long_Range_Radar_Sensor/1(Objects_Dectected_LRR[bool]) -> Object_Selection_Based_On_LRR_MRR_and_Camera SENSOR FUSION/1(Objects_Dectected_LRR[bool])
  Bus Selector/2 -> Object_Selection_Based_On_LRR_MRR_and_Camera SENSOR FUSION/11(Yaw_Angle_VUT[rad])  "<Yaw_Angle>"
  Bus Selector/1 -> Object_Selection_Based_On_LRR_MRR_and_Camera SENSOR FUSION/10(Heading_Angle_Road_under_VUT[deg])  "<Heating_Angle_Road_under_VUT[deg]>"
  Feedback_ADAS/1 -> Input_Maping/1(Feedback_ADAS)
  Feedback_Simulationsumgebung/1 -> Bus Selector/1, Input_Maping/2(Feedback_Simulationsumgebung)
  Input_Maping/1(Position_Global_VUT_Vector[m]) -> Front_Mid_Range_Radar_Sensor/1(Position_VUT_Vector[m]), Front_Long_Range_Radar_Sensor/1(Position_VUT_Vector[m])
  Input_Maping/2(Oriantation_VUT_Vector[rad]) -> Front_Mid_Range_Radar_Sensor/2(Oriantation_VUT_Vector[rad]), Front_Long_Range_Radar_Sensor/2(Oriantation_VUT_Vector[rad])
  Output_Mapint/1(Sensors_Output) -> Sensors_ADAS/1
  Front_Long_Range_Radar_Sensor/3(Angle_Horizontal_Vector_LRR[rad]) -> Object_Selection_Based_On_LRR_MRR_and_Camera SENSOR FUSION/3(Angle_Horizontal_Vector_LRR[rad])
  Front_Long_Range_Radar_Sensor/4(Positon_of_detected_Points_LRR[m]) -> convert_xy_2_st/1(Positon_of_detected_Points_LRR[m])
  convert_xy_2_st/1(T_Detected_Points_LRR[m]) -> Object_Selection_Based_On_LRR_MRR_and_Camera SENSOR FUSION/4(T_Detected_Points_LRR[m])
  Object_Selection_Based_On_LRR_MRR_and_Camera SENSOR FUSION/1(Sensors_Front_Out) -> Output_Mapint/1(Sensors_Front_Out)
  Input_Maping/3(Position_Fellows[m]) -> Front_Mid_Range_Radar_Sensor/3(Position_Fellows[m]), Front_Long_Range_Radar_Sensor/3(Position_Fellows[m])
  Input_Maping/4(Oriantation_Fellows[rad]) -> Front_Mid_Range_Radar_Sensor/4(Oriantation_Fellows[rad]), Front_Long_Range_Radar_Sensor/4(Oriantation_Fellows[rad])
  Front_Mid_Range_Radar_Sensor/4(Positon_of_detected_Points_MRR[m]) -> convert_xy_2_st1/1(Positon_of_detected_Points[m])
  Front_Mid_Range_Radar_Sensor/2(delta_s_Vector_MRR[m]) -> Object_Selection_Based_On_LRR_MRR_and_Camera SENSOR FUSION/6(delta_s_Vector_MRR[m])
  Front_Mid_Range_Radar_Sensor/3(Angle_Horizontal_Vector_MRR[rad]) -> Object_Selection_Based_On_LRR_MRR_and_Camera SENSOR FUSION/7(Angle_Horizontal_Vector_MRR[rad])
  Front_Mid_Range_Radar_Sensor/1(Objects_Dectected_MRR[bool]) -> Object_Selection_Based_On_LRR_MRR_and_Camera SENSOR FUSION/5(Objects_Dectected_MRR[bool])
  convert_xy_2_st1/1(T_Detected_Points[m]) -> Object_Selection_Based_On_LRR_MRR_and_Camera SENSOR FUSION/8(T_Detected_Points_MRR[m])
  Front_Long_Range_Radar_Sensor/2(delta_s_Vector_LRR[m]) -> Object_Selection_Based_On_LRR_MRR_and_Camera SENSOR FUSION/2(delta_s_Vector_LRR[m])
  [T_VP] -> Object_Selection_Based_On_LRR_MRR_and_Camera SENSOR FUSION/9(T_VUT[m])

== system PC_Simulator_Lib/ADAS/Unser_Interface_ADAS ==
  Feedback_ADAS : Inport
  Feedback_Simulationsumgebung : Inport  Port=2
  ACC_User_Interface : Subsystem
  Bus Creator : BusCreator
  Bus Creator1 : BusCreator  Inputs=3
  Bus Creator2 : BusCreator  Inputs=1
  Bus Creator3 : BusCreator  Inputs=1
  Bus Creator4 : BusCreator  Inputs=1
  Emergency_Brake : Subsystem
  Emergency_Steering : Subsystem
  Pilotiertes_Fahren : Subsystem
  UnserInterface_ADAS : Outport
  wires:
  Bus Creator/1 -> UnserInterface_ADAS/1  "UnserInterface_ADAS"
  Bus Creator1/1 -> Bus Creator/1  "ACC"
  ACC_User_Interface/1(ACC_State[bool]) -> Bus Creator1/1  "ACC_State"
  ACC_User_Interface/2(ACC_Set_Speed[m|s]) -> Bus Creator1/2  "ACC_Set_Speed[m|s]"
  ACC_User_Interface/3(ACC_Time_Gap_Mode[1-3]) -> Bus Creator1/3  "ACC_Time_Gap[s]"
  Feedback_Simulationsumgebung/1 -> Emergency_Steering/2(Feedback_Simulationsumgebung), Emergency_Brake/2(Feedback_Simulationsumgebung), Pilotiertes_Fahren/2(Feedback_Simulationsumgebung), ACC_User_Interface/2(Feedback_Simulationsumgebung)
  Bus Creator2/1 -> Bus Creator/2  "Pilotiertes_Fahren"
  Pilotiertes_Fahren/1(Pilotiertes_Fahren_State[bool]) -> Bus Creator2/1  "Pilotiertes_Fahren_State"
  Feedback_ADAS/1 -> Emergency_Steering/1(Feedback_ADAS), Emergency_Brake/1(Feedback_ADAS), Pilotiertes_Fahren/1(Feedback_ADAS), ACC_User_Interface/1(Feedback_ADAS)
  Bus Creator3/1 -> Bus Creator/3  "Emergency_Brake"
  Emergency_Brake/1(Emergency_Brake_State[bool]) -> Bus Creator3/1  "Emergency_Brake_State"
  Bus Creator4/1 -> Bus Creator/4  "Emergency_Steering"
  Emergency_Steering/1(Emergency_Steering_State[bool]) -> Bus Creator4/1  "Emergency_Steering_State"
